simulink model "working_ball_model_simulink"  (R2022b)
settings: Solver=VariableStepAuto  StartTime=0.0  StopTime=200  RelTol=1e-3
settings Model: PacingRate=1000  Creator=User  LastModifiedBy=User
settings SolverCC: ZeroCrossAlgorithm=Adaptive
settings DebuggingCC: IgnoredZcDiagnostic=none

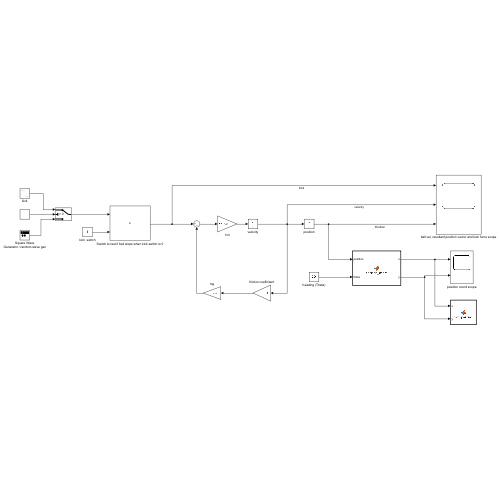
[thumbnail: Simulink's stored preview of the top-level diagram]
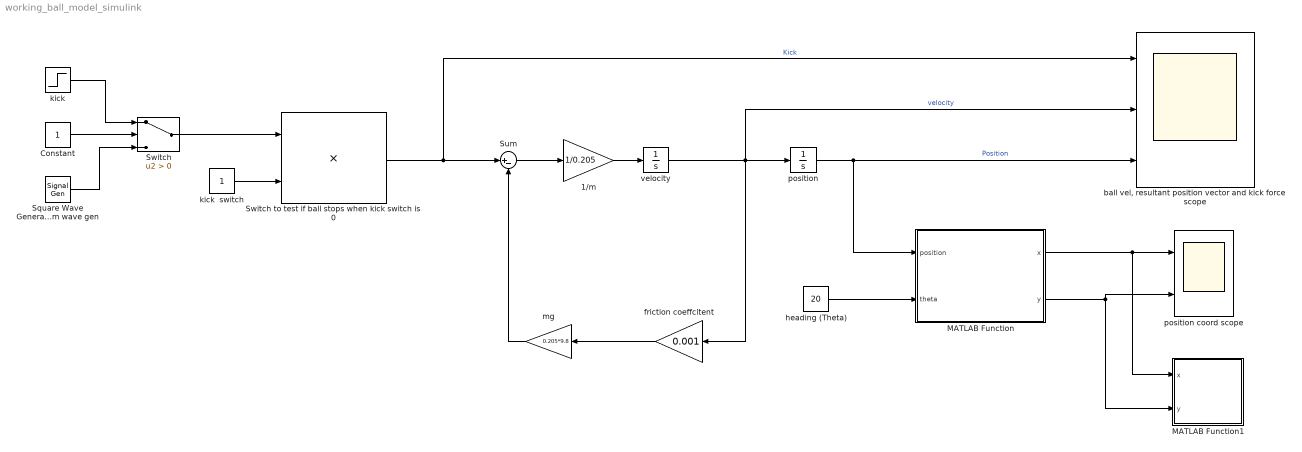
== system working_ball_model_simulink ==
  1/m : Gain  Gain=1/0.205
  Constant : Constant
  MATLAB Function : MATLAB Function  TreatAsAtomicUnit=on
  MATLAB Function1 : MATLAB Function  TreatAsAtomicUnit=on
  Square Wave Generator / random wave gen : SignalGenerator  WaveForm=random  Amplitude=5  Frequency=20
  Sum : Sum  Inputs=|+-
  Switch : Switch  Criteria=u2 > Threshold  SaturateOnIntegerOverflow=off  InputSameDT=off
  Switch to test if ball stops when kick switch is 0 : Product
  "ball vel, resultant position vector and kick force scope" : Scope  NumInputPorts=3
  friction coeffcitent : Gain  Gain=0.001
  heading (Theta) : Constant  Value=20
  kick : Step  Time=0.01  Before=5  After=0  SampleTime=0
  kick  switch : Constant
  mg : Gain  Gain=0.205*9.8
  position : Integrator
  position coord scope : Scope  NumInputPorts=2
  velocity : Integrator
  wires:
  1/m/1 -> velocity/1
  Sum/1 -> 1/m/1
  velocity/1 -> position/1, friction coeffcitent/1, "ball vel, resultant position vector and kick force scope"/2  "velocity"
  friction coeffcitent/1 -> mg/1
  mg/1 -> Sum/2
  position/1 -> "ball vel, resultant position vector and kick force scope"/3, MATLAB Function/1(position)  "Position"
  heading (Theta)/1 -> MATLAB Function/2(theta)
  MATLAB Function/1(x) -> MATLAB Function1/1(x), position coord scope/1
  MATLAB Function/2(y) -> position coord scope/2, MATLAB Function1/2(y)
  kick/1 -> Switch/1
  Constant/1 -> Switch/2
  Square Wave Generator / random wave gen/1 -> Switch/3
  Switch to test if ball stops when kick switch is 0/1 -> "ball vel, resultant position vector and kick force scope"/1, Sum/1  "Kick"
  Switch/1 -> Switch to test if ball stops when kick switch is 0/1
  kick  switch/1 -> Switch to test if ball stops when kick switch is 0/2

== matlab function working_ball_model_simulink/MATLAB Function ==
  data: position input; x output; theta input; y output
function [x,y] = position_coord(position, theta)

x = position*cos(theta);
y = position*sin(theta);

== matlab function working_ball_model_simulink/MATLAB Function1 ==
  data: x input; y input
function plot_position(x, y)
figure(1); clf; hold on; grid on; axis([-30,30,-30,30]);
plot(x,y,'Color','b','Marker','o');
